simulink model "DBZ_DiscreteTimeControl_first"  (R2023b)
settings: Solver=VariableStepAuto  StartTime=0.0  StopTime=100  RelTol=1e-3
values from neighbouring files (symbols this model uses):
  T = 0.2    [DBZ_DiscreteTimeControl_one.m]    (also in DBZ_DiscreteTimeControl_two.m = 0.01)
libraries: cstblocks x1
settings Model: Creator=Nezam Avaran  LastModifiedBy=Nezam Avaran

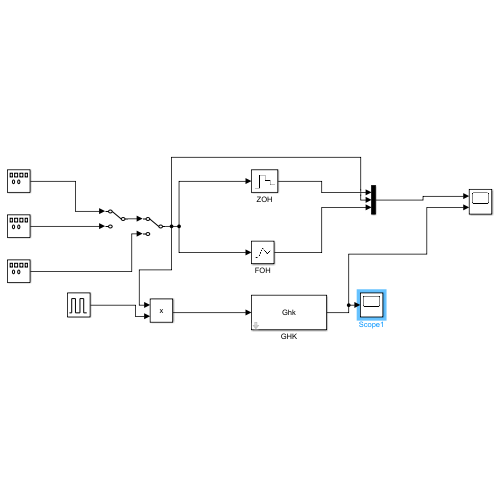
[thumbnail: Simulink's stored preview of the top-level diagram]
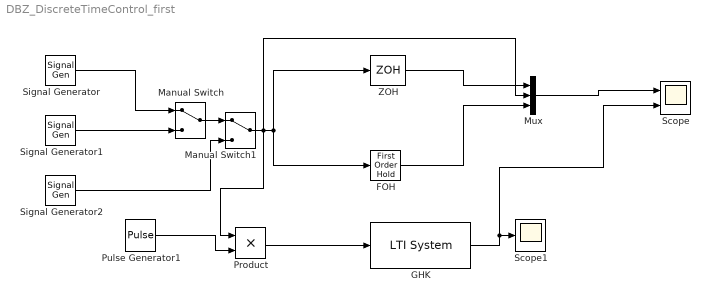
== system DBZ_DiscreteTimeControl_first ==
  FOH : FirstOrderHold  InitialOutput=T  ErrorTolerance=inf  AllowContinuousInput=on
  GHK : cstblocks/LTI System  sys=Ghk  IC=0  PadeOrder=0
  Manual Switch : ManualSwitch
  Manual Switch1 : ManualSwitch
  Mux : Mux  Inputs=3
  Product : Product
  Pulse Generator1 : DiscretePulseGenerator  PulseType=Time based  Amplitude=0.1/(0.001*T)  Period=T  PulseWidth=0.001
  Scope : Scope  NumInputPorts=2
  Scope1 : Scope
  Signal Generator : SignalGenerator  Amplitude=10  Units=rad/sec
  Signal Generator1 : SignalGenerator  WaveForm=square  Amplitude=10  Units=rad/sec
  Signal Generator2 : SignalGenerator  WaveForm=sawtooth  Amplitude=10  Units=rad/sec
  ZOH : ZeroOrderHold  SampleTime=T
  wires:
  Signal Generator/1 -> Manual Switch/1
  Signal Generator1/1 -> Manual Switch/2
  Signal Generator2/1 -> Manual Switch1/2
  Manual Switch/1 -> Manual Switch1/1
  Manual Switch1/1 -> Product/1, Mux/2, FOH/1, ZOH/1
  Mux/1 -> Scope/1
  FOH/1 -> Mux/3
  ZOH/1 -> Mux/1
  Pulse Generator1/1 -> Product/2
  Product/1 -> GHK/1
  GHK/1 -> Scope/2, Scope1/1
